simulink model "bms_f4"  (R2021a)
settings: Solver=FixedStepAuto  StartTime=0.0  StopTime=10.0  RelTol=1e-3  EnableMultiTasking=on
values from neighbouring files (symbols this model uses):
  CellCurrentLimitThreshold_Fault = 50    [fault_parameters.m]
  CellCurrentLimitThreshold_Warning = 20    [fault_parameters.m]
  CellTemperatureLimitThreshold_Fault = 65 + 273.15    (= 338.15)    [fault_parameters.m]
  CellTemperatureLimitThreshold_Warning = 50 + 273.15    (= 323.15)    [fault_parameters.m]
  CellVoltageLimitHigh_Fault = 4.25    [fault_parameters.m]
  CellVoltageLimitHigh_Warning = 4.21    [fault_parameters.m]
  CellVoltageLimitLow_Fault = 2.65    [fault_parameters.m]
  CellVoltageLimitLow_Warning = 2.70    (= 2.7)    [fault_parameters.m]
libraries: simulink x8
settings Model: Creator=miche  LastModifiedBy=miche
settings OptimizationCC: EnhancedBackFolding=on  PassReuseOutputArgsAs=Individual arguments  ZeroExternalMemoryAtStartup=off  ZeroInternalMemoryAtStartup=off  MaxStackSize=64  OptimizeBlockOrder=speed  DifferentSizesBufferReuse=on  OptimizationCustomize=off  EfficientTunableParamExpr=on
settings DebuggingCC: SignalInfNanChecking=warning  ParameterTunabilityLossMsg=error  AssertControl=DisableAll
settings HardwareCC: ProdBitPerPointer=32  ProdBitPerSizeT=32  ProdBitPerPtrDiffT=32  ProdLargestAtomicInteger=Long  ProdLargestAtomicFloat=Double  ProdWordSize=32  ProdHWDeviceType=ARM Compatible->ARM Cortex
settings SFSimCC: CompileTimeRecursionLimit=0  EnableRuntimeRecursion=off  MATLABDynamicMemAlloc=off
settings RTWCC: SystemTargetFile=ert.tlc  HardwareBoard=STM32F4-Discovery  TemplateMakefile=ert_default_tmf  Toolchain=GNU Tools for ARM Embedded Processors
settings CodeAppCC: ForceParamTrailComments=on  IgnoreCustomStorageClasses=off  OperatorAnnotations=on  SimulinkDataObjDesc=on  SFDataObjDesc=on  InsertBlockDesc=on
settings ERTTargetCC: CodeReplacementLibrary=ARM Cortex-M (Optimized)  ExtModeTransport=1  ExtModeMexFile=ext_serial_win32_comm

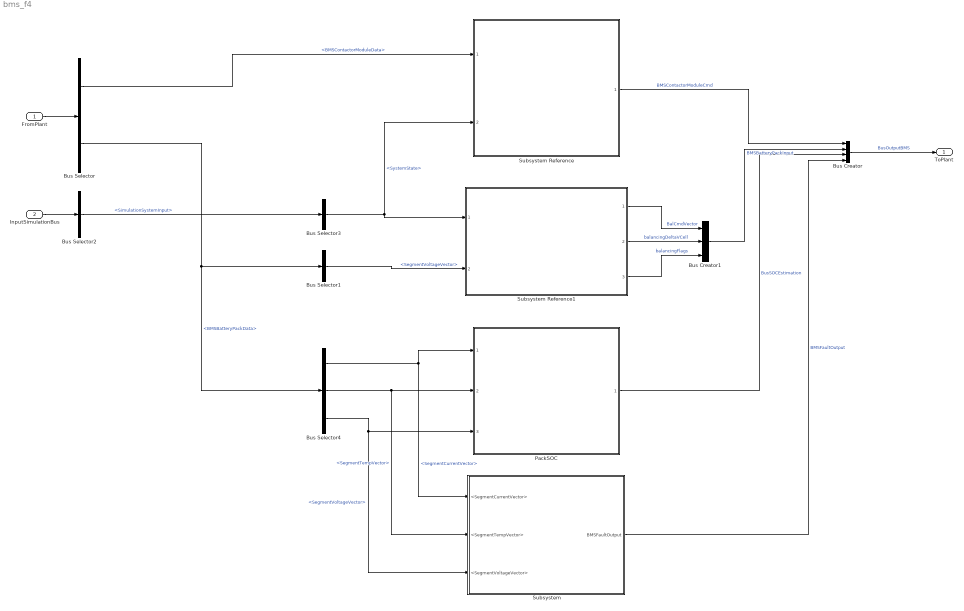
== system bms_f4 ==
  FromPlant : Inport  OutDataTypeStr=Bus: BusInputBMS
  InputSimulationBus : Inport  Port=2  OutDataTypeStr=Bus: BusSimulationInput
  Bus Creator : BusCreator  Inputs=4  OutDataTypeStr=Bus: BusOutputBMS
  Bus Creator1 : BusCreator  Inputs=3  OutDataTypeStr=Bus: BMSBatteryPackInput
  Bus Selector : BusSelector  OutputSignals=BMSContactorModuleData,BMSBatteryPackData
  Bus Selector1 : BusSelector  OutputSignals=SegmentVoltageVector
  Bus Selector2 : BusSelector  OutputSignals=SimulationSystemInput
  Bus Selector3 : BusSelector  OutputSignals=SystemState
  Bus Selector4 : BusSelector  OutputSignals=SegmentCurrentVector,SegmentTempVector,SegmentVoltageVector
  PackSOC : Subsystem  ReferencedSubsystem=PackSOC
  Subsystem : Subsystem
      mask Display: image('$imagefile'); % Use "Edit Image" on toolstrip to change.
  Subsystem Reference : Subsystem  ReferencedSubsystem=contactor_logic
  Subsystem Reference1 : Subsystem  ReferencedSubsystem=passive_balancing_logic
  ToPlant : Outport  OutDataTypeStr=Bus: BusOutputBMS
  wires:
  Subsystem Reference/1 -> Bus Creator/1  "BMSContactorModuleCmd"
  Subsystem Reference1/1 -> Bus Creator1/1  "BalCmdVector"
  Bus Creator1/1 -> Bus Creator/2  "BMSBatteryPackInput"
  Bus Creator/1 -> ToPlant/1  "BusOutputBMS"
  FromPlant/1 -> Bus Selector/1
  Bus Selector/1 -> Subsystem Reference/1  "<BMSContactorModuleData>"
  Bus Selector/2 -> Bus Selector4/1, Bus Selector1/1  "<BMSBatteryPackData>"
  Bus Selector1/1 -> Subsystem Reference1/2  "<SegmentVoltageVector>"
  InputSimulationBus/1 -> Bus Selector2/1
  Bus Selector2/1 -> Bus Selector3/1  "<SimulationSystemInput>"
  Bus Selector3/1 -> Subsystem Reference/2, Subsystem Reference1/1  "<SystemState>"
  Bus Selector4/1 -> PackSOC/1, Subsystem/1(<SegmentCurrentVector>)  "<SegmentCurrentVector>"
  Bus Selector4/3 -> Subsystem/3(<SegmentVoltageVector>), PackSOC/3  "<SegmentVoltageVector>"
  PackSOC/1 -> Bus Creator/3  "BusSOCEstimation"
  Bus Selector4/2 -> Subsystem/2(<SegmentTempVector>), PackSOC/2  "<SegmentTempVector>"
  Subsystem Reference1/2 -> Bus Creator1/2  "balancingDeltaVCell"
  Subsystem Reference1/3 -> Bus Creator1/3  "balancingFlags"
  Subsystem/1(BMSFaultOutput) -> Bus Creator/4  "BMSFaultOutput"

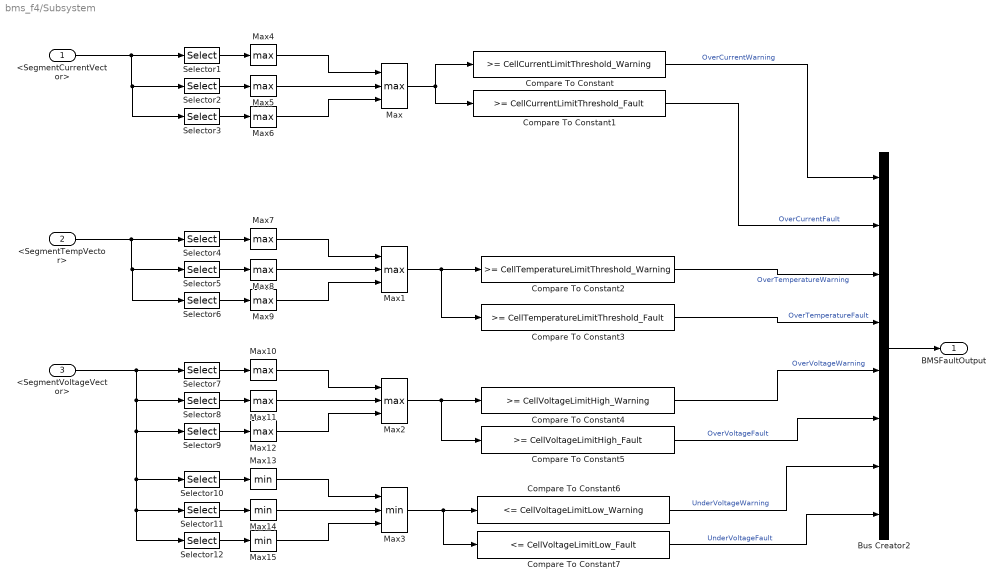
== system bms_f4/Subsystem ==
  <SegmentCurrentVector> : Inport
  <SegmentTempVector> : Inport  Port=2
  <SegmentVoltageVector> : Inport  Port=3
  Bus Creator2 : BusCreator  Inputs=8  OutDataTypeStr=Bus: BMSFaultOutput
  Compare To Constant : simulink/Logic and Bit Operations/Compare To Constant  relop=>=  const=CellCurrentLimitThreshold_Warning  OutDataTypeStr=boolean
  Compare To Constant1 : simulink/Logic and Bit Operations/Compare To Constant  relop=>=  const=CellCurrentLimitThreshold_Fault  OutDataTypeStr=boolean
  Compare To Constant2 : simulink/Logic and Bit Operations/Compare To Constant  relop=>=  const=CellTemperatureLimitThreshold_Warning  OutDataTypeStr=boolean
  Compare To Constant3 : simulink/Logic and Bit Operations/Compare To Constant  relop=>=  const=CellTemperatureLimitThreshold_Fault  OutDataTypeStr=boolean
  Compare To Constant4 : simulink/Logic and Bit Operations/Compare To Constant  relop=>=  const=CellVoltageLimitHigh_Warning  OutDataTypeStr=boolean
  Compare To Constant5 : simulink/Logic and Bit Operations/Compare To Constant  relop=>=  const=CellVoltageLimitHigh_Fault  OutDataTypeStr=boolean
  Compare To Constant6 : simulink/Logic and Bit Operations/Compare To Constant  relop=<=  const=CellVoltageLimitLow_Warning  OutDataTypeStr=boolean
  Compare To Constant7 : simulink/Logic and Bit Operations/Compare To Constant  relop=<=  const=CellVoltageLimitLow_Fault  OutDataTypeStr=boolean
  Max : MinMax  Function=max  Inputs=3
  Max1 : MinMax  Function=max  Inputs=3
  Max{4..12} (9 alike) : MinMax  Function=max
  Max13 : MinMax
  Max14 : MinMax
  Max15 : MinMax
  Max2 : MinMax  Function=max  Inputs=3
  Max3 : MinMax  Inputs=3
  Selector{1,4,7,10} (4 alike) : Selector  NumberOfDimensions=2  InputPortWidth=3  IndexOptions=Index vector (dialog),Index vector (dialog)  Indices=1,[1 2 3 4 5 6 7 8 9 10]  OutputSizes=1,1
  Selector{2,5,8,11} (4 alike) : Selector  NumberOfDimensions=2  InputPortWidth=3  IndexOptions=Index vector (dialog),Index vector (dialog)  Indices=2,[1 2 3 4 5 6 7 8 9 10]  OutputSizes=1,1
  Selector{3,6,9,12} (4 alike) : Selector  NumberOfDimensions=2  InputPortWidth=3  IndexOptions=Index vector (dialog),Index vector (dialog)  Indices=3,[1 2 3 4 5 6 7 8 9 10]  OutputSizes=1,1
  BMSFaultOutput : Outport
  wires:
  Compare To Constant2/1 -> Bus Creator2/3  "OverTemperatureWarning"
  Max3/1 -> Compare To Constant7/1, Compare To Constant6/1
  Bus Creator2/1 -> BMSFaultOutput/1
  Compare To Constant6/1 -> Bus Creator2/7  "UnderVoltageWarning"
  Max2/1 -> Compare To Constant5/1, Compare To Constant4/1
  Compare To Constant/1 -> Bus Creator2/1  "OverCurrentWarning"
  Compare To Constant5/1 -> Bus Creator2/6  "OverVoltageFault"
  Max1/1 -> Compare To Constant3/1, Compare To Constant2/1
  Max/1 -> Compare To Constant1/1, Compare To Constant/1
  Compare To Constant4/1 -> Bus Creator2/5  "OverVoltageWarning"
  Compare To Constant7/1 -> Bus Creator2/8  "UnderVoltageFault"
  Compare To Constant3/1 -> Bus Creator2/4  "OverTemperatureFault"
  Compare To Constant1/1 -> Bus Creator2/2  "OverCurrentFault"
  Selector2/1 -> Max5/1
  Selector1/1 -> Max4/1
  Selector3/1 -> Max6/1
  <SegmentCurrentVector>/1 -> Selector3/1, Selector2/1, Selector1/1
  Max4/1 -> Max/1
  Max5/1 -> Max/2
  Max6/1 -> Max/3
  Selector4/1 -> Max7/1
  <SegmentTempVector>/1 -> Selector6/1, Selector5/1, Selector4/1
  Selector5/1 -> Max8/1
  Selector6/1 -> Max9/1
  Max7/1 -> Max1/1
  Max9/1 -> Max1/3
  Max8/1 -> Max1/2
  Selector7/1 -> Max10/1
  Selector8/1 -> Max11/1
  Selector9/1 -> Max12/1
  Max10/1 -> Max2/1
  Max12/1 -> Max2/3
  Max11/1 -> Max2/2
  Selector10/1 -> Max13/1
  <SegmentVoltageVector>/1 -> Selector9/1, Selector12/1, Selector11/1, Selector10/1, Selector8/1, Selector7/1
  Selector11/1 -> Max14/1
  Selector12/1 -> Max15/1
  Max13/1 -> Max3/1
  Max15/1 -> Max3/3
  Max14/1 -> Max3/2
